simulink model "dashboard"  (R2022b)
settings: Solver=VariableStepAuto  StartTime=0.0  StopTime=inf  RelTol=1e-3
libraries: instrumentseriallib x2
settings Model: Creator=joseph  LastModifiedBy=joseph

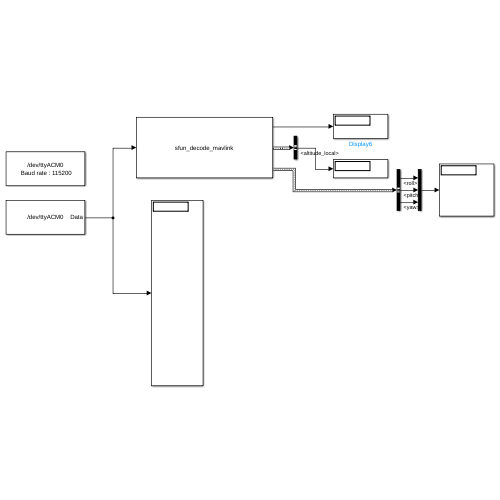
[thumbnail: Simulink's stored preview of the top-level diagram]
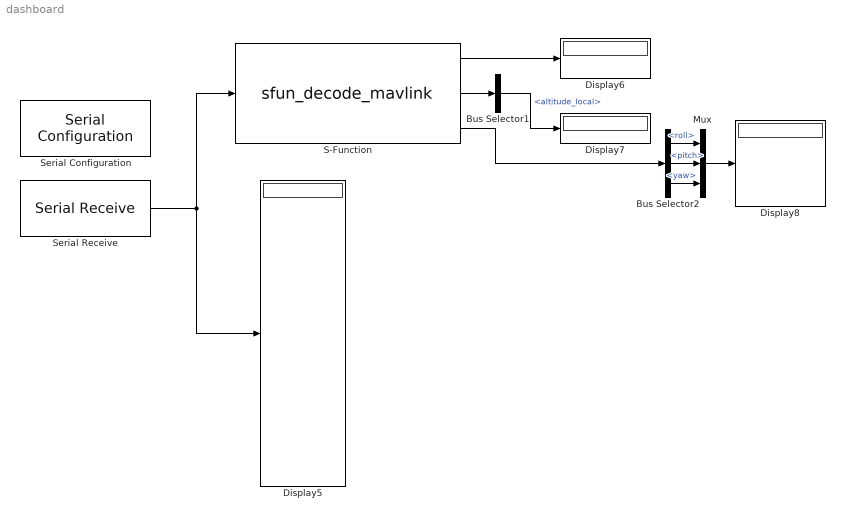
== system dashboard ==
  Bus Selector1 : BusSelector  OutputSignals=altitude_local
  Bus Selector2 : BusSelector  OutputSignals=roll,pitch,yaw
  Display{5..8} (4 alike) : Display
  Mux : Mux  Inputs=3
  S-Function : S-Function  FunctionName=sfun_decode_mavlink  SFunctionDeploymentMode=off  EnableBusSupport=off
  Serial Configuration : instrumentseriallib/Serial Configuration  Priority=-200000  PortSel=/dev/ttyACM0  Port=/dev/ttyACM0  ComPort=/dev/ttyACM0  BaudRate=115200  DataBits=8  Parity=none  StopBits=1  ByteOrder=little-endian  FlowControl=none  Timeout=10  SimulateUsing=Interpreted execution  BlockInModel=on  aMode=1
  Serial Receive : instrumentseriallib/Serial Receive  Priority=1  PortSel=/dev/ttyACM0  Port=/dev/ttyACM0  ComPort=/dev/ttyACM0  DataType=uint8  SaveDataType=uint8  ToggleHeader=off  Header=[]  ToggleTerminator=off  Terminator=<none>  CustomTerminator=[]  InputFormat=Column major  ToggleDataSize=on  DataSize=560  EnableBlockingMode=on  ActionDataUnavailable=Output last received value  ActionWhenDataUnavailable=Output last received value  CustomValue=0  SampleTime=0.01  SimulateUsing=Interpreted execution  BlockInModel=on  aMode=1
  wires:
  Serial Receive/1 -> Display5/1, S-Function/1
  S-Function/3 -> Bus Selector2/1
  S-Function/2 -> Bus Selector1/1
  S-Function/1 -> Display6/1
  Bus Selector1/1 -> Display7/1  "<altitude_local>"
  Bus Selector2/1 -> Mux/1  "<roll>"
  Bus Selector2/2 -> Mux/2  "<pitch>"
  Bus Selector2/3 -> Mux/3  "<yaw>"
  Mux/1 -> Display8/1
